simulink model "center_seeking_control"  (Simulink 3.00)
libraries: mathlib x9, reglib x4, execlib x2, logiclib x1, arclib x1

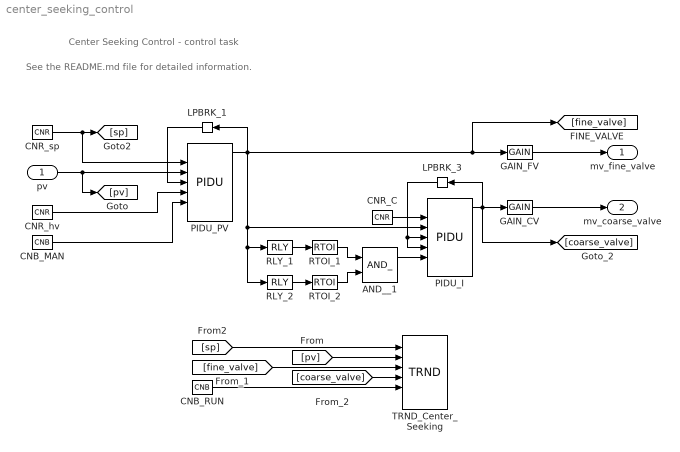
== system center_seeking_control ==
  note: See the README.md file for detailed information.
  note: Center Seeking Control - control task
  pv : Inport  Port=1
  AND__1 : logiclib/AND_
  CNB_MAN : mathlib/CNB  YCN=off
  CNB_RUN : mathlib/CNB  YCN=on
  CNR_C : mathlib/CNR  ycn=0.5
  CNR_hv : mathlib/CNR  ycn=0.1
  CNR_sp : mathlib/CNR  ycn=0
  GAIN_CV : mathlib/GAIN  k=0.8
  GAIN_FV : mathlib/GAIN  k=0.2
  LPBRK_1 : execlib/LPBRK  Orientation=left
  LPBRK_3 : execlib/LPBRK  Orientation=left
  PIDU_I : reglib/PIDU  irtype=2: I  RACT=on  k=1.0  ti=50  td=1  nd=10  b=1  c=0  tt=1  hilim=1  lolim=0  dz=0  icotype=1: Analog
  PIDU_PV : reglib/PIDU  irtype=7: PID  RACT=off  k=0.6  ti=4  td=1  nd=10  b=1  c=0  tt=1  hilim=1  lolim=0  dz=0  icotype=1: Analog
  RLY_1 : reglib/RLY  ep=0.45  en=0.25  ap=1  an=0  y0=0
  RLY_2 : reglib/RLY  ep=0.75  en=0.55  ap=0  an=1  y0=0
  RTOI_1 : mathlib/RTOI
  RTOI_2 : mathlib/RTOI
  TRND_Center_Seeking : arclib/TRND  n=4  l=1000  btype=8: Double  ptype1=1: Store  ptype2=1: Store  ptype3=1: Store  ptype4=1: Store  pfac=1  afac=0  arc=0  id=1  Title=Trend Title  timesrc=1
  mv_fine_valve : Outport  Port=1
  mv_coarse_valve : Outport  Port=2
  wires:
  AND__1/1 -> PIDU_I/6
  CNB_MAN/1 -> PIDU_PV/6
  CNB_RUN/1 -> TRND_Center_Seeking/5
  CNR_C/1 -> PIDU_I/2
  CNR_hv/1 -> PIDU_PV/5
  CNR_sp/1 -> [sp], PIDU_PV/2
  [pv] -> TRND_Center_Seeking/2
  [sp] -> TRND_Center_Seeking/1
  [fine_valve] -> TRND_Center_Seeking/3
  [coarse_valve] -> TRND_Center_Seeking/4
  GAIN_CV/1 -> mv_coarse_valve/1
  GAIN_FV/1 -> mv_fine_valve/1
  LPBRK_1/1 -> PIDU_PV/4
  LPBRK_3/1 -> PIDU_I/5, PIDU_I/4
  PIDU_I/1 -> GAIN_CV/1, [coarse_valve], LPBRK_3/1
  PIDU_PV/1 -> LPBRK_1/1, [fine_valve], GAIN_FV/1, PIDU_I/3, RLY_1/1, RLY_2/1
  RLY_1/1 -> RTOI_1/1
  RLY_2/1 -> RTOI_2/1
  RTOI_1/1 -> AND__1/1
  RTOI_2/1 -> AND__1/2
  pv/1 -> [pv], PIDU_PV/3
